simulink model "stepper_driver_example"  (R2020a)
settings: Solver=FixedStepAuto  StartTime=0.0  StopTime=inf  RelTol=1e-3  EnableMultiTasking=on
libraries: mbedblockslib x6
settings Model: SimulationMode=accelerator  SILPILModeSetting=veronly  ExtModeTrigDuration=10  Creator=pokpong.c  LastModifiedBy=szgno
settings SolverCC: PositivePriorityOrder=on
settings OptimizationCC: StrengthReduction=on  PassReuseOutputArgsAs=Individual arguments  ZeroExternalMemoryAtStartup=off  ZeroInternalMemoryAtStartup=off  MaxStackSize=64  OptimizeBlockOrder=speed  OptimizationPriority=Speed  OptimizationCustomize=off  MultiThreadedLoops=on  EfficientTunableParamExpr=on
settings DebuggingCC: ParameterTunabilityLossMsg=error
settings HardwareCC: ProdBitPerPointer=32  ProdBitPerSizeT=32  ProdBitPerPtrDiffT=32  ProdLargestAtomicInteger=Long  ProdLargestAtomicFloat=Double  ProdWordSize=32  ProdHWDeviceType=ARM Compatible->ARM Cortex
settings ModelReferenceCC: ModelReferenceNumInstancesAllowed=Single
settings SFSimCC: MATLABDynamicMemAlloc=off
settings RTWCC: SystemTargetFile=ert.tlc  HardwareBoard=STM32 Nucleo F411RE  TLCOptions=-aInlineSetEventsForThisBaseRateFcn=TLC_FALSE -aSuppressMultiTaskScheduler=TLC_FALSE -aRateBasedStepFcn=1  TemplateMakefile=ert_default_tmf  GenerateReport=on  Toolchain=GNU Tools for ARM Embedded Processors  IncludeHyperlinkInReport=on  LaunchReport=on  GenerateTraceInfo=on  GenerateTraceReport=on  GenerateTraceReportSl=on  GenerateTraceReportSf=on  GenerateTraceReportEml=on
settings CodeAppCC: ForceParamTrailComments=on  IgnoreCustomStorageClasses=off  OperatorAnnotations=on  SimulinkDataObjDesc=on  SFDataObjDesc=on  InsertBlockDesc=on
settings ERTTargetCC: SupportContinuousTime=on  ExtModeStaticAllocSize=2000

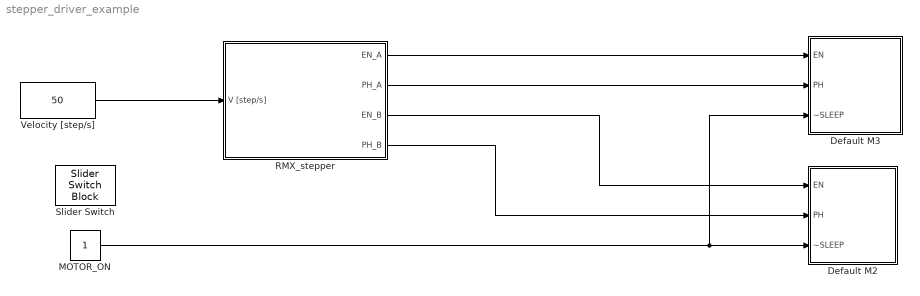
== system stepper_driver_example ==
  Default M2 : Subsystem
  Default M3 : Subsystem
  MOTOR_ON : Constant
  RMX_stepper : Subsystem  mask{i_coil=10, rev=off}
      mask prompts: i_coil "Duty Cycle [%]"; rev "Reverse Direction"
  Slider Switch : SliderSwitchBlock
      settings: Values={{'Off', 'On'}, [0 1]}
  Velocity [step/s] : Constant  Value=50
  wires:
  MOTOR_ON/1 -> Default M3/3(~SLEEP), Default M2/3(~SLEEP)
  RMX_stepper/1(EN_A) -> Default M3/1(EN)
  RMX_stepper/2(PH_A) -> Default M3/2(PH)
  RMX_stepper/3(EN_B) -> Default M2/1(EN)
  RMX_stepper/4(PH_B) -> Default M2/2(PH)
  Velocity [step/s]/1 -> RMX_stepper/1(V [step/s])

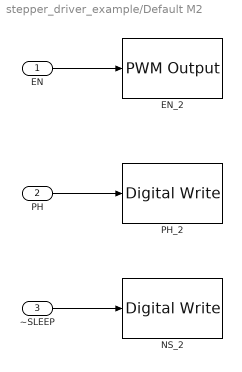
== system stepper_driver_example/Default M2 ==
  EN : Inport
  PH : Inport  Port=2
  ~SLEEP : Inport  Port=3
  EN_2 : mbedblockslib/PWM Output  Pin=PA_11  EnableInputFrequency=off  InitialFrequency=2000  InitialDutyCycle=50  NotificationType=None
      settings: SourceProductBaseCode=MICROBIT,NUCLEO,STMICRODIS
  NS_2 : mbedblockslib/Digital Write  Pin=PB_2  Direction=output
      settings: SourceProductBaseCode=MICROBIT,NUCLEO,STMICRODIS
  PH_2 : mbedblockslib/Digital Write  Pin=PC_7  Direction=output
      settings: SourceProductBaseCode=MICROBIT,NUCLEO,STMICRODIS
  wires:
  ~SLEEP/1 -> NS_2/1
  EN/1 -> EN_2/1
  PH/1 -> PH_2/1

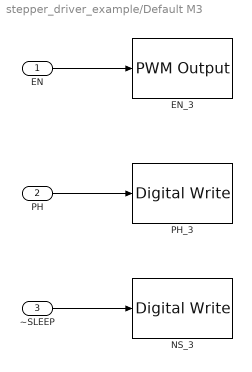
== system stepper_driver_example/Default M3 ==
  EN : Inport
  PH : Inport  Port=2
  ~SLEEP : Inport  Port=3
  EN_3 : mbedblockslib/PWM Output  Pin=PA_9  EnableInputFrequency=off  InitialFrequency=2000  InitialDutyCycle=50  NotificationType=None
      settings: SourceProductBaseCode=MICROBIT,NUCLEO,STMICRODIS
  NS_3 : mbedblockslib/Digital Write  Pin=PB_15  Direction=output
      settings: SourceProductBaseCode=MICROBIT,NUCLEO,STMICRODIS
  PH_3 : mbedblockslib/Digital Write  Pin=PB_10  Direction=output
      settings: SourceProductBaseCode=MICROBIT,NUCLEO,STMICRODIS
  wires:
  PH/1 -> PH_3/1
  ~SLEEP/1 -> NS_3/1
  EN/1 -> EN_3/1

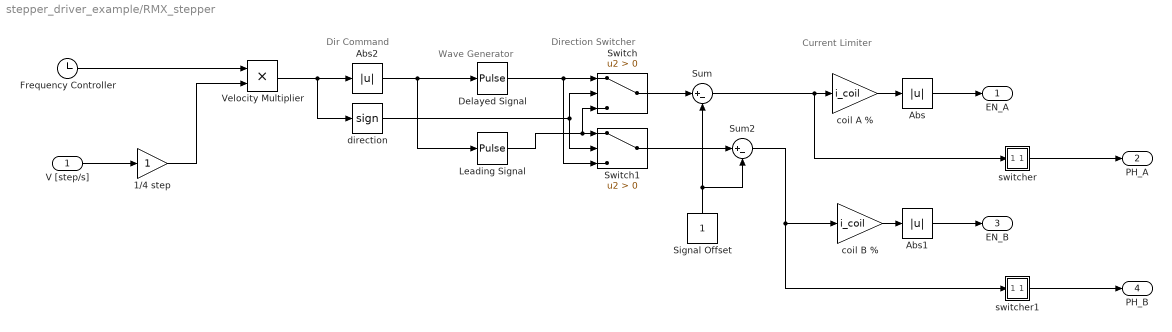
== system stepper_driver_example/RMX_stepper ==
  note: Direction Switcher
  note: Wave Generator
  note: Current Limiter
  note: Dir Command
  V [step/s] : Inport
  1/4 step : Gain
  Abs : Abs
  Abs1 : Abs
  Abs2 : Abs
  Delayed Signal : DiscretePulseGenerator  PulseType=Time based  TimeSource=Use external signal  Amplitude=2  Period=1  PulseWidth=50  PhaseDelay=1/4
  Frequency Controller : Clock
  Leading Signal : DiscretePulseGenerator  PulseType=Time based  TimeSource=Use external signal  Amplitude=2  Period=1  PulseWidth=50
  Signal Offset : Constant  SampleTime=0.001
  Sum : Sum  Inputs=|+-
  Sum2 : Sum  Inputs=|+-
  Switch : Switch  Criteria=u2 > Threshold
  Switch1 : Switch  Criteria=u2 > Threshold
  Velocity Multiplier : Product
  coil A % : Gain  Gain=i_coil
  coil B % : Gain  Gain=i_coil
  direction : Signum
  switcher : Subsystem
  switcher1 : Subsystem
  EN_A : Outport
  PH_A : Outport  Port=2
  EN_B : Outport  Port=3
  PH_B : Outport  Port=4
  wires:
  Sum/1 -> coil A %/1, switcher/1(I)
  Sum2/1 -> coil B %/1, switcher1/1(I)
  Abs/1 -> EN_A/1
  Abs1/1 -> EN_B/1
  Leading Signal/1 -> Switch/3, Switch1/1
  Switch/1 -> Sum/1
  Velocity Multiplier/1 -> direction/1, Abs2/1
  Delayed Signal/1 -> Switch/1, Switch1/3
  Switch1/1 -> Sum2/1
  Abs2/1 -> Leading Signal/1, Delayed Signal/1
  Signal Offset/1 -> Sum2/2, Sum/2
  direction/1 -> Switch/2, Switch1/2
  Frequency Controller/1 -> Velocity Multiplier/1
  switcher/1(O) -> PH_A/1
  switcher1/1(O) -> PH_B/1
  coil A %/1 -> Abs/1
  coil B %/1 -> Abs1/1
  V [step/s]/1 -> 1/4 step/1
  1/4 step/1 -> Velocity Multiplier/2

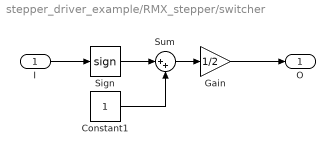
== system stepper_driver_example/RMX_stepper/switcher ==
  I : Inport
  Constant1 : Constant
  Gain : Gain  Gain=1/2
  Sign : Signum
  Sum : Sum  Inputs=|++
  O : Outport
  wires:
  Sign/1 -> Sum/1
  Constant1/1 -> Sum/2
  Gain/1 -> O/1
  Sum/1 -> Gain/1
  I/1 -> Sign/1

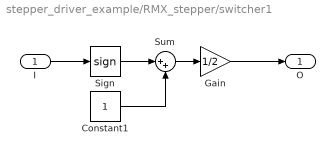
== system stepper_driver_example/RMX_stepper/switcher1 ==
  I : Inport
  Constant1 : Constant
  Gain : Gain  Gain=1/2
  Sign : Signum
  Sum : Sum  Inputs=|++
  O : Outport
  wires:
  I/1 -> Sign/1
  Sum/1 -> Gain/1
  Gain/1 -> O/1
  Constant1/1 -> Sum/2
  Sign/1 -> Sum/1
